simulink model "ysw3_45"  (R2014a)
settings: Solver=ode45  StartTime=0.0  StopTime=10.0  RelTol=1e-3
settings Model: Creator=Administrator  LastModifiedBy=Administrator

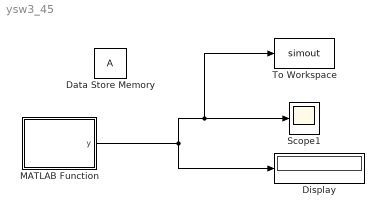
== system ysw3_45 ==
  Data Store Memory : DataStoreMemory  ReadBeforeWriteMsg=warning  WriteAfterWriteMsg=warning  WriteAfterReadMsg=warning  InitialValue=25  OutDataTypeStr=double
  Display : Display
  MATLAB Function : MATLAB Function  TreatAsAtomicUnit=on
  Scope1 : Scope
      settings: TimeRange=10
  To Workspace : ToWorkspace  VariableName=simout  SaveFormat=Timeseries  SampleTime=-1
  wires:
  MATLAB Function/1(y) -> Display/1, To Workspace/1, Scope1/1

== matlab function ysw3_45/MATLAB Function ==
  data: y output; A data_store_memory
function y = fcn
%#codegen
global A;
A = A+1;
y = A;
